simulink library "Lib_DQTrans_dqe2abcProductT"  (R2021a)
settings: Solver=VariableStepAuto  StartTime=0.0  StopTime=10.0  RelTol=1e-3
undefined symbols (not defined in the file): C_SQRT3
libraries: Lib_DQTrans_dqe2dqs x1
settings Model: Creator=30610  LastModifiedBy=30610

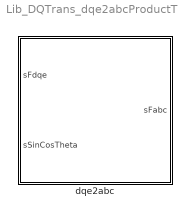
== system Lib_DQTrans_dqe2abcProductT ==
  dqe2abc : Subsystem

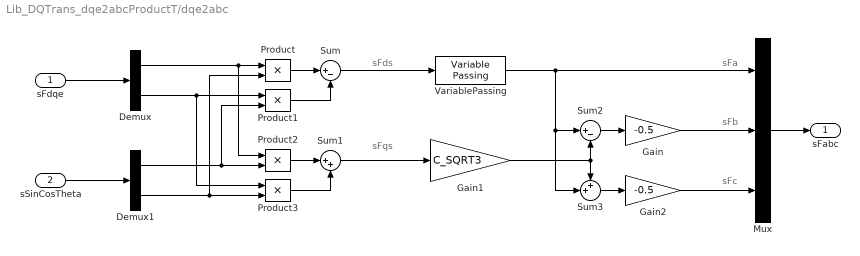
== system Lib_DQTrans_dqe2abcProductT/dqe2abc ==
  note: sFc
  note: sFb
  note: sFa
  note: sFqs
  note: sFds
  sFdqe : Inport
  sSinCosTheta : Inport  Port=2
  Demux : Demux  Outputs=2
  Demux1 : Demux  Outputs=2
  Gain : Gain  Gain=-0.5
  Gain1 : Gain  Gain=C_SQRT3
  Gain2 : Gain  Gain=-0.5
  Mux : Mux  Inputs=3
  Product{,1..3} (4 alike) : Product  RndMeth=Zero
  Sum : Sum  Inputs=|+-
  Sum1 : Sum  Inputs=|++
  Sum2 : Sum  Inputs=|+-
  Sum3 : Sum  Inputs=++|
  VariablePassing : Lib_DQTrans_dqe2dqs/dqe2dqs/Variable Passing  SystemSampleTime=-1  VariantActivationTime=update diagram  Latency=0  AutoFrameSizeCalculation=off
  sFabc : Outport  VectorParamsAs1DForOutWhenUnconnected=off
  wires:
  sSinCosTheta/1 -> Demux1/1
  Demux/1 -> Product2/1, Product/1
  Demux/2 -> Product3/1, Product1/1
  Sum/1 -> VariablePassing/1
  Product2/1 -> Sum1/1
  Sum1/1 -> Gain1/1
  Product1/1 -> Sum/2
  Product3/1 -> Sum1/2
  sFdqe/1 -> Demux/1
  Product/1 -> Sum/1
  Demux1/1 -> Product1/2, Product2/2
  Demux1/2 -> Product/2, Product3/2
  Gain1/1 -> Sum3/1, Sum2/2
  VariablePassing/1 -> Mux/1, Sum3/2, Sum2/1
  Sum3/1 -> Gain2/1
  Sum2/1 -> Gain/1
  Gain/1 -> Mux/2
  Gain2/1 -> Mux/3
  Mux/1 -> sFabc/1
